simulink model "BP_example"  (Simulink 7.3)
settings: Solver=ode45  StartTime=0.0  StopTime=250  MaxStep=.01  MinStep=.0001  RelTol=1e-6  AbsTol=1e-6
PreLoadFcn:
  | [D,SigD,h,Sigh] = eval([bdroot,'Params']); % Pendulum Parameters
  | load([bdroot,'TestObjParams.mat']); % Test object parameters [m,I,C,KD,Th0,ThBias]
  | load([bdroot,'Data.mat']); % experimental data
values from neighbouring files (symbols this model uses):
  C = 0.00230784823238    [BP_exampleTestObjParams.mat]
  D = mean([moiexpdata(1) moiexpdata(3)])    [BP_exampleParams.m]    (also in calculateInertiaLinearApprox.m = 0.343)
  h = mean([moiexpdata(5) moiexpdata(7)])    [BP_exampleParams.m]    (also in calculateInertiaLinearApprox.m = 1.873)
  I = 0.393650417341    [BP_exampleTestObjParams.mat]    (also in calculateInertiaLinearApprox.m = (m*g*D^2)/(4*h*wn^2))
  KD = 0.00974463743363    [BP_exampleTestObjParams.mat]
  m = 1.54122    [BP_exampleTestObjParams.mat]    (also in calculateInertiaLinearApprox.m = m_indoorHull)
  Th0 = 0.220510213373    [BP_exampleTestObjParams.mat]
  ThBias = -0.363451181564    [BP_exampleTestObjParams.mat]
settings Model: Creator=mjardin  LastModifiedBy=mjardin  SimulationMode=accelerator
settings DataIOCC: LimitDataPoints=off
settings OptimizationCC: InitFltsAndDblsToZero=on
settings DebuggingCC: SaveWithParameterizedLinksMsg=none
settings GRTTargetCC: TargetFcnLib=ansi_tfl_tmw.mat

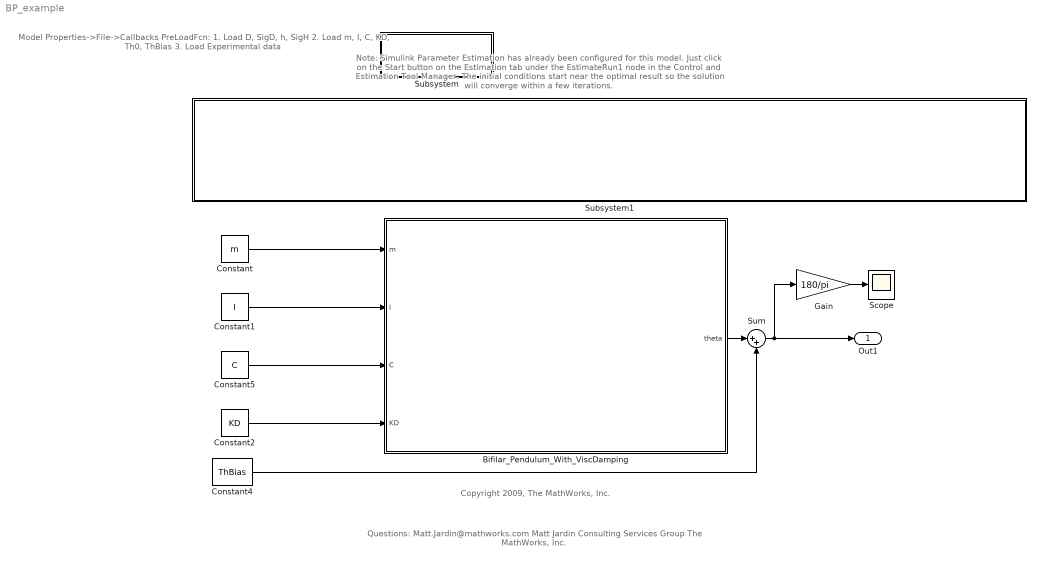
== system BP_example ==
  note: Model Properties->File->Callbacks
      | PreLoadFcn:
      |     1. Load D, SigD, h, SigH
      |     2. Load m, I, C, KD, Th0, ThBias
      |     3. Load Experimental data
  note: Copyright 2009, The MathWorks, Inc.
  note: Note: Simulink Parameter Estimation has already been configured
      | for this model. Just click on the Start button on the Estimation tab
      | under the EstimateRun1 node in the Control and Estimation Tool
      | Manager. The initial conditions start near the optimal result so
      | the solution will converge within a few iterations.
  note: Questions: Matt.Jardin@mathworks.com
      | Matt Jardin
      | Consulting Services Group
      | The MathWorks, Inc.
  Bifilar_Pendulum_With_ViscDamping : Subsystem  mask(Bifilar Pendulum Simulation){D=D, SigD=0, h=h, Sigh=0, SigTh=0, ThSeed=0, TH0_THBIAS=Th0-ThBias}
      mask prompts: D "Wire Displacement (D, meters)"; SigD "D Uncertainty (SigD, meters)"; h "Wire Height (h, meters)"; Sigh "h Uncertainty (Sigh, meters)"; SigTh "Theta Uncertainty (SigTh, radians)"; ThSeed "Theta Random Seed"; TH0_THBIAS "Initial Angular Displacement"
      mask help: This block simulates the response of a Bifilar Pendulum to an initial angular displacement. The parameters of the pendulum may be entered in the Mask Dialog.
      mask Help: No help yet.
      mask Display:
      | image(imread('inertiaexperimentcartoon_b.jpg'));
      | port_label('input',1,'mass')
      | port_label('input',2,'Moment of Inertia')
      | port_label('input',3','C, Viscous Damping Parameter')
      | port_label('input',4,'KD, Square-Law Damping Parameter')
      | port_label('output',1,'\theta','texmode','on');
  Constant : Constant  Value=m  OutDataType=sfix(16)  OutScaling=2^0
  Constant1 : Constant  Value=I  OutDataType=sfix(16)  OutScaling=2^0
  Constant2 : Constant  Value=KD  OutDataType=sfix(16)  OutScaling=2^0
  Constant4 : Constant  Value=ThBias  OutDataType=sfix(16)  OutScaling=2^0
  Constant5 : Constant  Value=C  OutDataType=sfix(16)  OutScaling=2^0
  Gain : Gain  Gain=180/pi  ParameterDataType=sfix(16)  ParameterScaling=2^0  OutDataType=sfix(16)  OutScaling=2^0
  Scope : Scope
      settings: TimeRange=250  YMin=-60  YMax=20
  Subsystem : Subsystem
      settings: OpenFcn=speload([bdroot,'EstPrj.mat'],['Project - ', bdroot], 'EstimateRun1')
      mask Display: text(0.5,0.5,sprintf('Double-Click\nto Run\nParameter Estimation'),'horizontalAlignment','center','verticalAlignment','middle')
  Subsystem1 : Subsystem
      mask Display: image(imread('BP_equation.jpg'))
  Sum : Sum  Inputs=|++  OutDataType=sfix(16)  OutScaling=2^0
  Out1 : Outport  OutDataType=sfix(16)  OutScaling=2^0
  wires:
  Constant/1 -> Bifilar_Pendulum_With_ViscDamping/1(m)
  Constant1/1 -> Bifilar_Pendulum_With_ViscDamping/2(I)
  Constant2/1 -> Bifilar_Pendulum_With_ViscDamping/4(KD)
  Bifilar_Pendulum_With_ViscDamping/1(theta) -> Sum/1
  Constant4/1 -> Sum/2
  Gain/1 -> Scope/1
  Sum/1 -> Out1/1, Gain/1
  Constant5/1 -> Bifilar_Pendulum_With_ViscDamping/3(C)

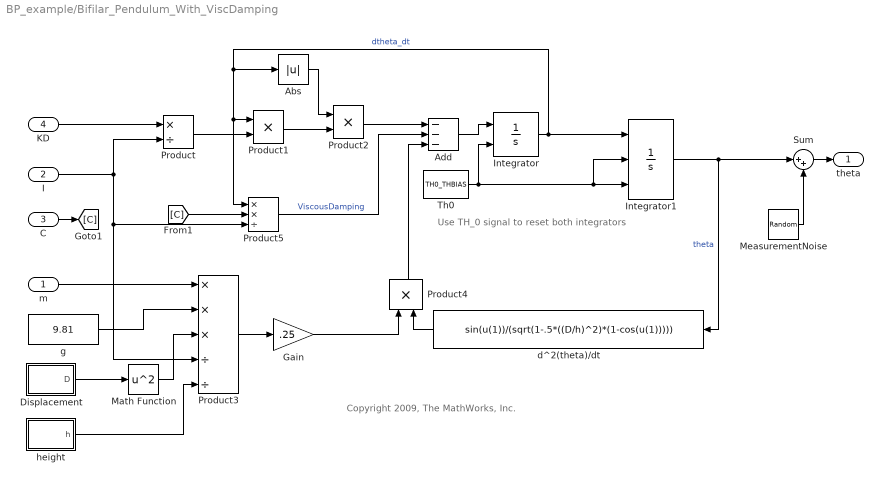
== system BP_example/Bifilar_Pendulum_With_ViscDamping ==
  note: Use TH_0 signal to
      | reset both integrators
  note: Copyright 2009, The MathWorks, Inc.
  m : Inport  OutDataType=sfix(16)  OutScaling=2^0
  I : Inport  Port=2  OutDataType=sfix(16)  OutScaling=2^0
  C : Inport  Port=3  OutDataType=sfix(16)  OutScaling=2^0
  KD : Inport  Port=4  OutDataType=sfix(16)  OutScaling=2^0
  Abs : Abs
  Add : Sum  Inputs=---  OutDataType=sfix(16)  OutScaling=2^-10
  Displacement : Subsystem
  Gain : Gain  Gain=.25  ParameterDataType=sfix(16)  ParameterScaling=2^0  OutDataType=sfix(16)  OutScaling=2^0
  Integrator : Integrator  ExternalReset=either
  Integrator1 : Integrator  ExternalReset=either  InitialConditionSource=external
  Math Function : Math  Operator=square  OutDataType=sfix(16)  OutScaling=2^0  SaturateOnIntegerOverflow=on
  MeasurementNoise : RandomNumber  Variance=SigTh*SigTh  Seed=ThSeed  SampleTime=0
  Product : Product  Inputs=*/  OutDataType=sfix(16)  OutScaling=2^0  RndMeth=Zero
  Product1 : Product  Inputs=**  OutDataType=sfix(16)  OutScaling=2^0  RndMeth=Zero
  Product2 : Product  Inputs=**  OutDataType=sfix(16)  OutScaling=2^0  RndMeth=Zero
  Product3 : Product  Inputs=***//  OutDataType=sfix(16)  OutScaling=2^0  RndMeth=Zero
  Product4 : Product  Inputs=**  OutDataType=sfix(16)  OutScaling=2^0  RndMeth=Zero
  Product5 : Product  Inputs=**/  OutDataType=sfix(16)  OutScaling=2^0  RndMeth=Zero
  Sum : Sum  Inputs=|++  OutDataType=sfix(16)  OutScaling=2^0
  Th0 : Constant  Value=TH0_THBIAS  OutDataType=sfix(16)  OutScaling=2^0
  d^2(theta)/dt : Fcn  Expr=sin(u(1))/(sqrt(1-.5*((D/h)^2)*(1-cos(u(1)))))
  g : Constant  Value=9.81  OutDataType=sfix(16)  OutScaling=2^0
  height : Subsystem
  theta : Outport  OutDataType=sfix(16)  OutScaling=2^0
  wires:
  Th0/1 -> Integrator/2, Integrator1/2, Integrator1/3
  Gain/1 -> Product4/1
  d^2(theta)/dt/1 -> Product4/2
  Product3/1 -> Gain/1
  height/1(h) -> Product3/5
  Math Function/1 -> Product3/3
  g/1 -> Product3/2
  m/1 -> Product3/1
  Displacement/1(D) -> Math Function/1
  Integrator1/1 -> d^2(theta)/dt/1, Sum/1  "theta"
  Product2/1 -> Add/1
  Add/1 -> Integrator/1
  Integrator/1 -> Integrator1/1, Abs/1, Product1/1, Product5/1  "dtheta_dt"
  Abs/1 -> Product2/1
  Product1/1 -> Product2/2
  Product/1 -> Product1/2
  I/1 -> Product/2, Product3/4, Product5/3
  KD/1 -> Product/1
  C/1 -> [C]
  [C] -> Product5/2
  Product5/1 -> Add/2  "ViscousDamping"
  Product4/1 -> Add/3
  Sum/1 -> theta/1
  MeasurementNoise/1 -> Sum/2

== system BP_example/Subsystem ==

== system BP_example/Subsystem1 ==
  note: This subsystem intentionally left blank.

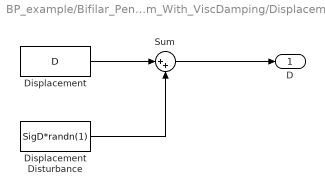
== system BP_example/Bifilar_Pendulum_With_ViscDamping/Displacement ==
  Displacement : Constant  Value=D  OutDataType=sfix(16)  OutScaling=2^0
  Displacement Disturbance : Constant  Value=SigD*randn(1)  OutDataType=sfix(16)  OutScaling=2^0
  Sum : Sum  Inputs=|++  OutDataType=sfix(16)  OutScaling=2^0
  D : Outport  OutDataType=sfix(16)  OutScaling=2^0
  wires:
  Displacement Disturbance/1 -> Sum/2
  Sum/1 -> D/1
  Displacement/1 -> Sum/1

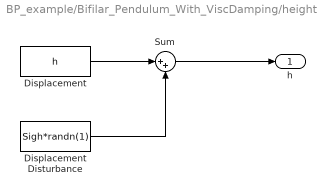
== system BP_example/Bifilar_Pendulum_With_ViscDamping/height ==
  Displacement : Constant  Value=h  OutDataType=sfix(16)  OutScaling=2^0
  Displacement Disturbance : Constant  Value=Sigh*randn(1)  OutDataType=sfix(16)  OutScaling=2^0
  Sum : Sum  Inputs=|++  OutDataType=sfix(16)  OutScaling=2^0
  h : Outport  OutDataType=sfix(16)  OutScaling=2^0
  wires:
  Displacement/1 -> Sum/1
  Sum/1 -> h/1
  Displacement Disturbance/1 -> Sum/2
